simulink library "urarm_simulink"  (R2013a)
settings: Solver=ode45  StartTime=0.0  StopTime=10.0  RelTol=1e-3
values from neighbouring files (symbols this model uses):
  URARM_HANDLE = URArm    [hwinit_urarm.m]
settings Model: Creator=Fankai  LastModifiedBy=Fankai

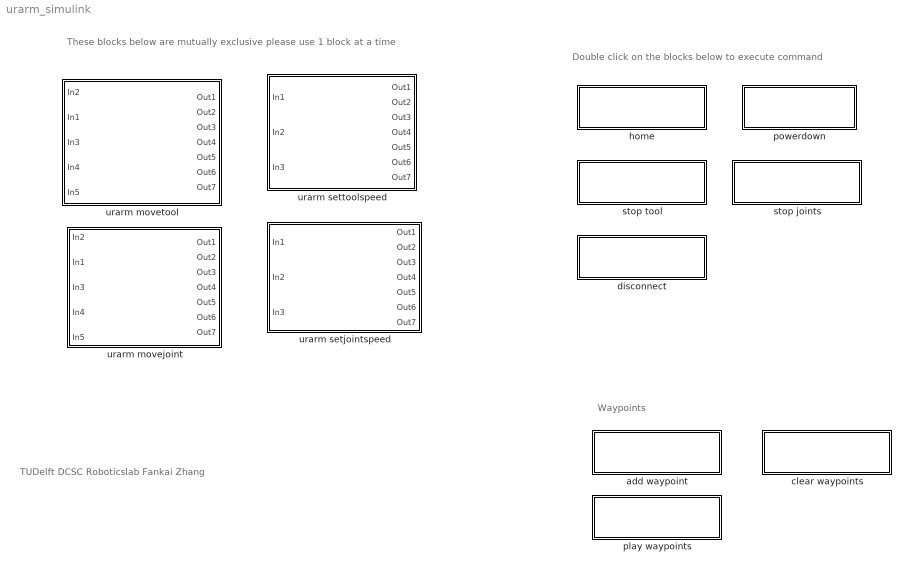
== system urarm_simulink ==
  note: Waypoints
  note: Double click on the blocks below to execute command
  note: TUDelft DCSC Roboticslab
      | Fankai Zhang
  note: These blocks below are
      | mutually exclusive
      | please use 1 block at a time
  add waypoint : Subsystem
      settings: OpenFcn=|
      | if exist('URARM_HANDLE','var') && ~isempty(URARM_HANDLE)
      | URARM_HANDLE.appendWaypoint();
      | end
      mask Display: fprintf('double click me\n to add current waypoint')
  clear waypoints : Subsystem
      settings: OpenFcn=|
      | if exist('URARM_HANDLE','var') && ~isempty(URARM_HANDLE)
      | URARM_HANDLE.clearWaypoints();
      | end
      mask Display: fprintf('double click me\n to clear all waypoints')
  disconnect : Subsystem
      settings: OpenFcn=|
      | if exist('URARM_HANDLE','var') && ~isempty(URARM_HANDLE)
      | URARM_HANDLE.fclose();
      | end
      mask Display: fprintf('double click me\n to disconnect')
  home : Subsystem
      settings: OpenFcn=|
      | if exist('URARM_HANDLE','var') && ~isempty(URARM_HANDLE)
      | URARM_HANDLE.home();
      | end
      mask Display: fprintf('double click me\n to return to home pose')
  play waypoints : Subsystem
      settings: OpenFcn=|
      | if exist('URARM_HANDLE','var') && ~isempty(URARM_HANDLE)
      | URARM_HANDLE.playWaypoints();
      | end
      mask Display: fprintf('double click me\n to play waypoints')
  powerdown : Subsystem
      settings: OpenFcn=|
      | if exist('URARM_HANDLE','var') && ~isempty(URARM_HANDLE)
      | URARM_HANDLE.powerdown();
      | end
      mask Display: fprintf('double click me\n to powerdown urarm')
  stop joints : Subsystem
      settings: OpenFcn=|
      | if exist('URARM_HANDLE','var') && ~isempty(URARM_HANDLE)
      | URARM_HANDLE.stopJoints();
      | end
      mask Display: fprintf('double click me\n to stop joints')
  stop tool : Subsystem
      settings: OpenFcn=|
      | if exist('URARM_HANDLE','var') && ~isempty(URARM_HANDLE)
      | URARM_HANDLE.stopTool();
      | end
      mask Display: fprintf('double click me\n to stop tool')
  urarm movejoint : Subsystem  mask{Ts=0}
      mask prompts: Ts "SampleTime"
  urarm movetool : Subsystem  mask{Ts=0}
      mask prompts: Ts "SampleTime"
  urarm setjointspeed : Subsystem  mask{Ts=0}
      mask prompts: Ts "SampleTime"
  urarm settoolspeed : Subsystem  mask{Ts=0}
      mask prompts: Ts "SampleTime"

== system urarm_simulink/add waypoint ==

== system urarm_simulink/clear waypoints ==

== system urarm_simulink/disconnect ==

== system urarm_simulink/home ==

== system urarm_simulink/play waypoints ==

== system urarm_simulink/powerdown ==

== system urarm_simulink/stop joints ==

== system urarm_simulink/stop tool ==

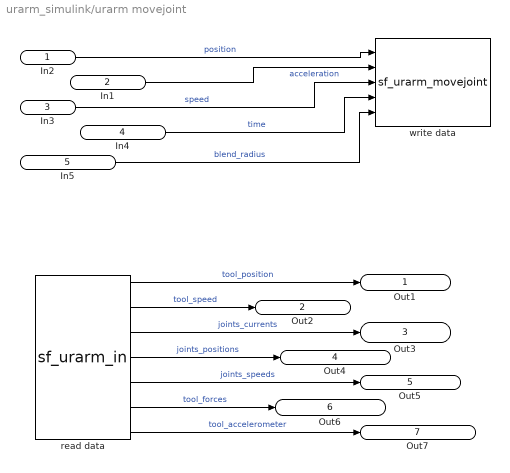
== system urarm_simulink/urarm movejoint ==
  In2 : Inport
  In1 : Inport  Port=2
  In3 : Inport  Port=3
  In4 : Inport  Port=4
  In5 : Inport  Port=5
  read data : M-S-Function  FunctionName=sf_urarm_in  Parameters=URARM_HANDLE
  write data : M-S-Function  FunctionName=sf_urarm_movejoint  Parameters=URARM_HANDLE,Ts
  Out1 : Outport
  Out2 : Outport  Port=2
  Out3 : Outport  Port=3
  Out4 : Outport  Port=4
  Out5 : Outport  Port=5
  Out6 : Outport  Port=6
  Out7 : Outport  Port=7
  wires:
  In2/1 -> write data/1  "position"
  In1/1 -> write data/2  "acceleration"
  In3/1 -> write data/3  "speed"
  read data/1 -> Out1/1  "tool_position"
  read data/2 -> Out2/1  "tool_speed"
  read data/3 -> Out3/1  "joints_currents"
  read data/4 -> Out4/1  "joints_positions"
  read data/5 -> Out5/1  "joints_speeds"
  read data/6 -> Out6/1  "tool_forces"
  read data/7 -> Out7/1  "tool_accelerometer"
  In4/1 -> write data/4  "time"
  In5/1 -> write data/5  "blend_radius"

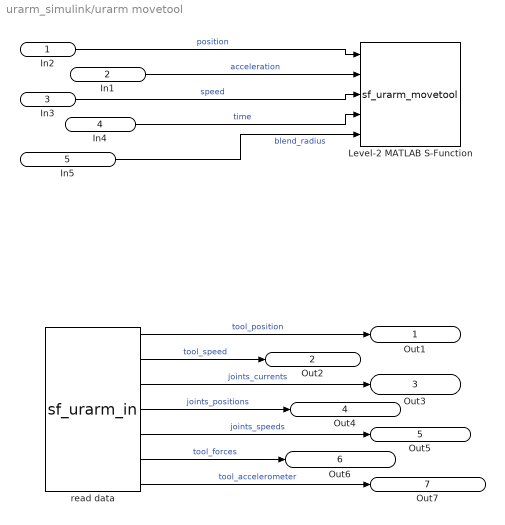
== system urarm_simulink/urarm movetool ==
  In2 : Inport
  In1 : Inport  Port=2
  In3 : Inport  Port=3
  In4 : Inport  Port=4
  In5 : Inport  Port=5
  Level-2 MATLAB S-Function : M-S-Function  FunctionName=sf_urarm_movetool  Parameters=URARM_HANDLE,Ts
  read data : M-S-Function  FunctionName=sf_urarm_in  Parameters=URARM_HANDLE
  Out1 : Outport
  Out2 : Outport  Port=2
  Out3 : Outport  Port=3
  Out4 : Outport  Port=4
  Out5 : Outport  Port=5
  Out6 : Outport  Port=6
  Out7 : Outport  Port=7
  wires:
  In2/1 -> Level-2 MATLAB S-Function/1  "position"
  In1/1 -> Level-2 MATLAB S-Function/2  "acceleration"
  read data/1 -> Out1/1  "tool_position"
  read data/2 -> Out2/1  "tool_speed"
  read data/3 -> Out3/1  "joints_currents"
  read data/4 -> Out4/1  "joints_positions"
  read data/5 -> Out5/1  "joints_speeds"
  read data/6 -> Out6/1  "tool_forces"
  read data/7 -> Out7/1  "tool_accelerometer"
  In3/1 -> Level-2 MATLAB S-Function/3  "speed"
  In4/1 -> Level-2 MATLAB S-Function/4  "time"
  In5/1 -> Level-2 MATLAB S-Function/5  "blend_radius"

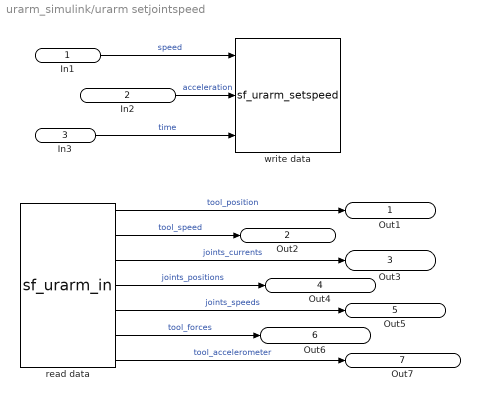
== system urarm_simulink/urarm setjointspeed ==
  In1 : Inport
  In2 : Inport  Port=2
  In3 : Inport  Port=3
  read data : M-S-Function  FunctionName=sf_urarm_in  Parameters=URARM_HANDLE
  write data : M-S-Function  FunctionName=sf_urarm_setspeed  Parameters=URARM_HANDLE,Ts
  Out1 : Outport
  Out2 : Outport  Port=2
  Out3 : Outport  Port=3
  Out4 : Outport  Port=4
  Out5 : Outport  Port=5
  Out6 : Outport  Port=6
  Out7 : Outport  Port=7
  wires:
  In1/1 -> write data/1  "speed"
  In2/1 -> write data/2  "acceleration"
  In3/1 -> write data/3  "time"
  read data/1 -> Out1/1  "tool_position"
  read data/2 -> Out2/1  "tool_speed"
  read data/3 -> Out3/1  "joints_currents"
  read data/4 -> Out4/1  "joints_positions"
  read data/5 -> Out5/1  "joints_speeds"
  read data/6 -> Out6/1  "tool_forces"
  read data/7 -> Out7/1  "tool_accelerometer"

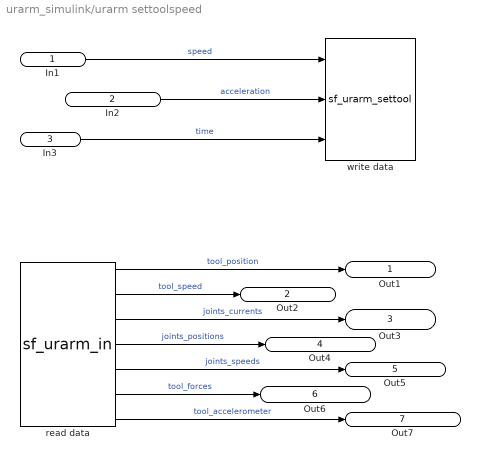
== system urarm_simulink/urarm settoolspeed ==
  In1 : Inport
  In2 : Inport  Port=2
  In3 : Inport  Port=3
  read data : M-S-Function  FunctionName=sf_urarm_in  Parameters=URARM_HANDLE
  write data : M-S-Function  FunctionName=sf_urarm_settool  Parameters=URARM_HANDLE,Ts
  Out1 : Outport
  Out2 : Outport  Port=2
  Out3 : Outport  Port=3
  Out4 : Outport  Port=4
  Out5 : Outport  Port=5
  Out6 : Outport  Port=6
  Out7 : Outport  Port=7
  wires:
  In1/1 -> write data/1  "speed"
  In2/1 -> write data/2  "acceleration"
  In3/1 -> write data/3  "time"
  read data/1 -> Out1/1  "tool_position"
  read data/2 -> Out2/1  "tool_speed"
  read data/3 -> Out3/1  "joints_currents"
  read data/4 -> Out4/1  "joints_positions"
  read data/5 -> Out5/1  "joints_speeds"
  read data/6 -> Out6/1  "tool_forces"
  read data/7 -> Out7/1  "tool_accelerometer"
